simulink model "Assembly_union"  (R2020a)
settings: Solver=VariableStepAuto  StartTime=0.0  StopTime=inf  RelTol=1e-3
model workspace: external: MATLAB File A:\Usuarios\TATTO PC\Desktop\univesidad\Procesamiento video y audio\proyecto 6 intelingencia artificial\Assembly3_DataFile.m (data not in the file)
undefined symbols (not defined in the file or in its folder): smiData, X, Y, Z
libraries: neural x563, sm_lib x153, nesl_utility x4, dspstat3 x3, audiosources x1, simulink x1, dspxfrm3 x1
(part 4 of 36)

== system Assembly_union/Subsystem/Custom Neural Network6/Layer 6 ==
  "a{5} " : Inport  PortDimensions=70
      mask Display: e = 0.06;c1 = [120 230 180]/255;c2 = ([120 230 180]+0)/(256+128);c3 = ([120 230 180]+128)/(256+128);patch([0 1 1 0],[0 0 1 1],c1);patch([0 1 1 1-e 1-e 0+e],[0 0 1 1-e 0+e 0+e],c2);patch([0 0 1 1-e 0+e 0+e],[0 1 1 1-e 1-e 0+e],c3);plot([0 1 1 0 0],[0 0 1 1 0]);
  Delays 1 : Subsystem
      mask Display: e = 0.06;c1 = [120 150 230]/255;c2 = ([120 150 230]+0)/383;c3 = ([120 150 230]+128)/383;patch([0 1 1 0],[0 0 1 1],c1);patch([0 1 1 1-e 1-e 0+e],[0 0 1 1-e 0+e 0+e],c2);patch([0 0 1 1-e 0+e 0+e],[0 1 1 1-e 1-e 0+e],c3);plot([0 1 1 0 0],[0 0 1 1 0]);disp('0');
  "LW{6,5}" : Subsystem
      mask Display: e = 0.06;c1 = [120 150 230]/255;c2 = ([120 150 230]+0)/383;c3 = ([120 150 230]+128)/383;patch([0 1 1 0],[0 0 1 1],c1);patch([0 1 1 1-e 1-e 0+e],[0 0 1 1-e 0+e 0+e],c2);patch([0 0 1 1-e 0+e 0+e],[0 1 1 1-e 1-e 0+e],c3);plot([0 1 1 0 0],[0 0 1 1 0]);disp('W');
  "b{6}" : Constant  Value=[-1.485003387606178559821046292199753224849700927734375;1.4578215715256430673463228231412358582019805908203125;-1.3893651088165828166864912418532185256481170654296875;1.360850145432328961447865367517806589603424072265625;-1.3163944869522321567956169019453227519989013671875;1.2790831565414564341409686676342971622943878173828125;-1.2301069748957143001888425715151242911815643310546875;-1.2053186311808909980669568540179170668125152587890625;-1.119571343264250895543909791740588843822479248046875;-1.105184198547311869020859376178123056888580322265625;1.0496333853723898155152483013807795941829681396484375;1.0079878762454252960623080070945434272289276123046875;-0.98533438913372239920107631405699066817760467529296875;-0.94027001026555623308667009041528217494487762451171875;-0.8726319445384718154201664219726808369159698486328125;-0.85683744760427982267714241970679722726345062255859375;-0.807565898785896241207638013293035328388214111328125;0.77004429336715407572455660556443035602569580078125;0.71850134366528506379978580298484303057193756103515625;-0.647167461466730653540935236378572881221771240234375;-0.592447199662568646516547232749871909618377685546875;0.59251503759554313699453587105381302535533905029296875;-0.536368947826048714233593273092992603778839111328125;-0.5162879618890394706198776475503109395503997802734375;0.44502670176876180097025326176662929356098175048828125;-0.411594605501536758840330776365590281784534454345703125;-0.385216068976885761543371700099669396877288818359375;0.32933495686654923328973154639243148267269134521484375;0.30167834932332515673891748519963584840297698974609375;0.23611842292874019033632748687523417174816131591796875;0.1826912311398599941814069325118907727301120758056640625;-0.145968008454668396467468483024276793003082275390625;-0.10534177126921299982864610456090304069221019744873046875;0.06018886059545865141462428482554969377815723419189453125;0.007770730586208964181527125703041747328825294971466064453125;-0.003037900210818963477044096777035520062781870365142822265625;-0.050253621911659558663121316612887312658131122589111328125;0.09786422466005463560723143245922983624041080474853515625;0.1510481711326792375604810558797908015549182891845703125;-0.1959526938701692533317810784865287132561206817626953125;-0.2351624924981109698851611256031901575624942779541015625;-0.277950698490396330697649318608455359935760498046875;-0.336603419162789518903622365542105399072170257568359375;-0.35305899148826125344413640050333924591541290283203125;-0.413619138650432704995552057880559004843235015869140625;-0.444163369013349740299645418417640030384063720703125;0.484800773696828446457374184319633059203624725341796875;0.55997085323872630713282205761061049997806549072265625;0.5889112097013391444733088064822368323802947998046875;0.6266854932690610890944071798003278672695159912109375;0.66414649891511590151793598124640993773937225341796875;0.70284249294120770823468546950607560575008392333984375;0.748702178371122517575031451997347176074981689453125;0.80946782172921671882903638106654398143291473388671875;-0.84566429400031228880152411875315010547637939453125;-0.88906859934408632994973231689073145389556884765625;-0.90484521568163334137580022797919809818267822265625;-0.97417279264519651693632340538897551596164703369140625;-1.023583515821328671080436834017746150493621826171875;1.0530542658285824142438968920032493770122528076171875;-1.091398208237234879192101288936100900173187255859375;1.141249173995749988108627803740091621875762939453125;-1.1619243888892019089809082288411445915699005126953125;-1.2241454031893457266022551266360096633434295654296875;1.2750005254271881138805611044517718255519866943359375;1.32597692828655322472286570700816810131072998046875;1.3199231160172217869330779649317264556884765625;1.404688225611195218078819380025379359722137451171875;1.44054888145474624394637430668808519840240478515625;-1.483986405440906874986239927238784730434417724609375]
      mask Display: e = 0.06;c1 = [120 150 230]/255;c2 = ([120 150 230]+0)/383;c3 = ([120 150 230]+128)/383;patch([0 1 1 0],[0 0 1 1],c1);patch([0 1 1 1-e 1-e 0+e],[0 0 1 1-e 0+e 0+e],c2);patch([0 0 1 1-e 0+e 0+e],[0 1 1 1-e 1-e 0+e],c3);plot([0 1 1 0 0],[0 0 1 1 0]);disp('b');
  netsum : Sum  Inputs=2  InputSameDT=on  SaturateOnIntegerOverflow=on  OutDataTypeStr=Inherit: Same as first input
      mask Display: e = 0.06;c1 = [120 150 230]/255;c2 = ([120 150 230]+0)/383;c3 = ([120 150 230]+128)/383;patch([0 1 1 0],[0 0 1 1],c1);patch([0 1 1 1-e 1-e 0+e],[0 0 1 1-e 0+e 0+e],c2);patch([0 0 1 1-e 0+e 0+e],[0 1 1 1-e 1-e 0+e],c3);plot([0 1 1 0 0],[0 0 1 1 0]);disp('+');
  tansig : neural/Transfer Functions/tansig
  "a{6}" : Outport  InitialOutput=[0;0;0;0;0;0;0;0;0;0;0;0;0;0;0;0;0;0;0;0;0;0;0;0;0;0;0;0;0;0;0;0;0;0;0;0;0;0;0;0;0;0;0;0;0;0;0;0;0;0;0;0;0;0;0;0;0;0;0;0;0;0;0;0;0;0;0;0;0;0]
      mask Display: e = 0.06;c1 = [120 230 180]/255;c2 = ([120 230 180]+0)/(256+128);c3 = ([120 230 180]+128)/(256+128);patch([0 1 1 0],[0 0 1 1],c1);patch([0 1 1 1-e 1-e 0+e],[0 0 1 1-e 0+e 0+e],c2);patch([0 0 1 1-e 0+e 0+e],[0 1 1 1-e 1-e 0+e],c3);plot([0 1 1 0 0],[0 0 1 1 0]);
  wires:
  "a{5} "/1 -> Delays 1/1("p{6}")
  Delays 1/1("pd{6,5}") -> "LW{6,5}"/1("ad{6,5}")
  "LW{6,5}"/1("lz{6,5}") -> netsum/1
  "b{6}"/1 -> netsum/2
  netsum/1 -> tansig/1
  tansig/1 -> "a{6}"/1

== system Assembly_union/Subsystem/Custom Neural Network6/Layer 7 ==
  "a{6} " : Inport  PortDimensions=70
      mask Display: e = 0.06;c1 = [120 230 180]/255;c2 = ([120 230 180]+0)/(256+128);c3 = ([120 230 180]+128)/(256+128);patch([0 1 1 0],[0 0 1 1],c1);patch([0 1 1 1-e 1-e 0+e],[0 0 1 1-e 0+e 0+e],c2);patch([0 0 1 1-e 0+e 0+e],[0 1 1 1-e 1-e 0+e],c3);plot([0 1 1 0 0],[0 0 1 1 0]);
  Delays 1 : Subsystem
      mask Display: e = 0.06;c1 = [120 150 230]/255;c2 = ([120 150 230]+0)/383;c3 = ([120 150 230]+128)/383;patch([0 1 1 0],[0 0 1 1],c1);patch([0 1 1 1-e 1-e 0+e],[0 0 1 1-e 0+e 0+e],c2);patch([0 0 1 1-e 0+e 0+e],[0 1 1 1-e 1-e 0+e],c3);plot([0 1 1 0 0],[0 0 1 1 0]);disp('0');
  "LW{7,6}" : Subsystem
      mask Display: e = 0.06;c1 = [120 150 230]/255;c2 = ([120 150 230]+0)/383;c3 = ([120 150 230]+128)/383;patch([0 1 1 0],[0 0 1 1],c1);patch([0 1 1 1-e 1-e 0+e],[0 0 1 1-e 0+e 0+e],c2);patch([0 0 1 1-e 0+e 0+e],[0 1 1 1-e 1-e 0+e],c3);plot([0 1 1 0 0],[0 0 1 1 0]);disp('W');
  "b{7}" : Constant  Value=[-1.4767621523240166414581153730978257954120635986328125;1.444049296004457527686781759257428348064422607421875;-1.4013145988464714708499059270252473652362823486328125;1.3335134565628778968715550945489667356014251708984375;1.3236197336460235884914027337799780070781707763671875;1.27579077866800094653854102944023907184600830078125;-1.21593386784343948647801880724728107452392578125;1.178120321207556830955809346050955355167388916015625;-1.12775361173192489872008081874810159206390380859375;1.078399371995239608423844401841051876544952392578125;-1.0560677697311307010608061318635009229183197021484375;1.0272419780436761183040061951032839715480804443359375;0.99828915385229344270356932611321099102497100830078125;-0.8858404721323822617051746419747360050678253173828125;-0.8576324002365949272785883295000530779361724853515625;0.8292697266285691259923851248458959162235260009765625;-0.8083178375879727095565385752706788480281829833984375;0.7069678528848524212691017964971251785755157470703125;-0.691934107202713644113600821583531796932220458984375;-0.62273911879922361212180703660123981535434722900390625;-0.61509936217620875265055246927659027278423309326171875;0.57882003721991981404215721340733580291271209716796875;0.539682981503778247400759937590919435024261474609375;-0.4993444993130979892015375298797152936458587646484375;0.469344644639037744671128393747494556009769439697265625;0.4214914724469507323334482862264849245548248291015625;-0.37938438865782397879655718497815541923046112060546875;-0.304543847702456293990991298414883203804492950439453125;0.284100250478663551856328695066622458398342132568359375;0.2391032035570020142234426430150051601231098175048828125;-0.1971118230385970060414280169425182975828647613525390625;-0.1768708078998612320820171817103982903063297271728515625;0.11242682486000869779285693539350177161395549774169921875;-0.06773328044365271860538513237770530395209789276123046875;0.01283256275473169949474794293564627878367900848388671875;0.052509615656154202956162890814084676094353199005126953125;0.056595446575947082334945292814154527150094509124755859375;0.0957661037569482453957192547022714279592037200927734375;0.1710599168838210226706308958455338142812252044677734375;-0.2004174313203110902037451523938216269016265869140625;0.2335509297283305529813191014909534715116024017333984375;0.310312095338587445869649172891513444483280181884765625;0.305696289894037409595739518408663570880889892578125;-0.36359794360045449845841858405037783086299896240234375;0.40952848771876404487812806110014207661151885986328125;0.438142211964403560653380509393173269927501678466796875;-0.53602802650183123400751128428964875638484954833984375;-0.5537352484590680745668578310869634151458740234375;0.5633847814036225809530833430471830070018768310546875;-0.60758518515698900497312706647790037095546722412109375;0.67224387508036897997953929007053375244140625;0.7521169924806463402688905262039043009281158447265625;-0.75404805176073186334662068475154228508472442626953125;0.78505703476111332594911118576419539749622344970703125;0.84022623832228882090333854648633860051631927490234375;0.89421096481471218364589503835304640233516693115234375;0.92810077829095971591044644810608588159084320068359375;-0.9541226123161259398131051057134754955768585205078125;1.008752849302839482703575413324870169162750244140625;-1.0517509919543404084407711707171984016895294189453125;1.0948916566899244973143368042656220495700836181640625;-1.122592887192439103927199539612047374248504638671875;-1.173968638316350787675901301554404199123382568359375;-1.213892733483060926147345526260323822498321533203125;1.2715677661036901557878309176885522902011871337890625;1.3291196102867590678187070807325653731822967529296875;-1.3539816759775289423117783371708355844020843505859375;-1.4025819142239408510164366816752590239048004150390625;1.4116364927836217990630984786548651754856109619140625;1.501802361522918349834299078793264925479888916015625]
      mask Display: e = 0.06;c1 = [120 150 230]/255;c2 = ([120 150 230]+0)/383;c3 = ([120 150 230]+128)/383;patch([0 1 1 0],[0 0 1 1],c1);patch([0 1 1 1-e 1-e 0+e],[0 0 1 1-e 0+e 0+e],c2);patch([0 0 1 1-e 0+e 0+e],[0 1 1 1-e 1-e 0+e],c3);plot([0 1 1 0 0],[0 0 1 1 0]);disp('b');
  netsum : Sum  Inputs=2  InputSameDT=on  SaturateOnIntegerOverflow=on  OutDataTypeStr=Inherit: Same as first input
      mask Display: e = 0.06;c1 = [120 150 230]/255;c2 = ([120 150 230]+0)/383;c3 = ([120 150 230]+128)/383;patch([0 1 1 0],[0 0 1 1],c1);patch([0 1 1 1-e 1-e 0+e],[0 0 1 1-e 0+e 0+e],c2);patch([0 0 1 1-e 0+e 0+e],[0 1 1 1-e 1-e 0+e],c3);plot([0 1 1 0 0],[0 0 1 1 0]);disp('+');
  tansig : neural/Transfer Functions/tansig
  "a{7}" : Outport  InitialOutput=[0;0;0;0;0;0;0;0;0;0;0;0;0;0;0;0;0;0;0;0;0;0;0;0;0;0;0;0;0;0;0;0;0;0;0;0;0;0;0;0;0;0;0;0;0;0;0;0;0;0;0;0;0;0;0;0;0;0;0;0;0;0;0;0;0;0;0;0;0;0]
      mask Display: e = 0.06;c1 = [120 230 180]/255;c2 = ([120 230 180]+0)/(256+128);c3 = ([120 230 180]+128)/(256+128);patch([0 1 1 0],[0 0 1 1],c1);patch([0 1 1 1-e 1-e 0+e],[0 0 1 1-e 0+e 0+e],c2);patch([0 0 1 1-e 0+e 0+e],[0 1 1 1-e 1-e 0+e],c3);plot([0 1 1 0 0],[0 0 1 1 0]);
  wires:
  "a{6} "/1 -> Delays 1/1("p{7}")
  Delays 1/1("pd{7,6}") -> "LW{7,6}"/1("ad{7,6}")
  "LW{7,6}"/1("lz{7,6}") -> netsum/1
  "b{7}"/1 -> netsum/2
  netsum/1 -> tansig/1
  tansig/1 -> "a{7}"/1

== system Assembly_union/Subsystem/Custom Neural Network6/Layer 8 ==
  "a{7} " : Inport  PortDimensions=70
      mask Display: e = 0.06;c1 = [120 230 180]/255;c2 = ([120 230 180]+0)/(256+128);c3 = ([120 230 180]+128)/(256+128);patch([0 1 1 0],[0 0 1 1],c1);patch([0 1 1 1-e 1-e 0+e],[0 0 1 1-e 0+e 0+e],c2);patch([0 0 1 1-e 0+e 0+e],[0 1 1 1-e 1-e 0+e],c3);plot([0 1 1 0 0],[0 0 1 1 0]);
  Delays 1 : Subsystem
      mask Display: e = 0.06;c1 = [120 150 230]/255;c2 = ([120 150 230]+0)/383;c3 = ([120 150 230]+128)/383;patch([0 1 1 0],[0 0 1 1],c1);patch([0 1 1 1-e 1-e 0+e],[0 0 1 1-e 0+e 0+e],c2);patch([0 0 1 1-e 0+e 0+e],[0 1 1 1-e 1-e 0+e],c3);plot([0 1 1 0 0],[0 0 1 1 0]);disp('0');
  "LW{8,7}" : Subsystem
      mask Display: e = 0.06;c1 = [120 150 230]/255;c2 = ([120 150 230]+0)/383;c3 = ([120 150 230]+128)/383;patch([0 1 1 0],[0 0 1 1],c1);patch([0 1 1 1-e 1-e 0+e],[0 0 1 1-e 0+e 0+e],c2);patch([0 0 1 1-e 0+e 0+e],[0 1 1 1-e 1-e 0+e],c3);plot([0 1 1 0 0],[0 0 1 1 0]);disp('W');
  "b{8}" : Constant  Value=[1.4870503804997989849567829878651537001132965087890625;-1.3951167688820780288239120636717416346073150634765625;-1.327618360170772948691819692612625658512115478515625;1.306601799763808191556790916365571320056915283203125;1.2663434339955046414871731030871160328388214111328125;1.190710745246216450965448530041612684726715087890625;-1.146077751003579781041707974509336054325103759765625;1.1207008038467944910365758914849720895290374755859375;-1.076304867027505718368729503708891570568084716796875;-1.0124811514544884705202321129036135971546173095703125;0.99231961835159199214473346728482283651828765869140625;-0.94089816984124585719229116875794716179370880126953125;-0.87244570582967828631382189996656961739063262939453125;0.8277766961789716493314017498050816357135772705078125;0.780486675323220691069536769646219909191131591796875;-0.7615131860318140599730440953862853348255157470703125;-0.68486451279397864144726781887584365904331207275390625;0.62709947678303412654798876246786676347255706787109375;-0.64579718495621174501053474159562028944492340087890625;0.55706567783365013024621248405310325324535369873046875;-0.5049344991792865666724310358404181897640228271484375;0.472820940457257699041093701453064568340778350830078125;0.429017711810034507724509467152529396116733551025390625;0.3446190033229241667100950508029200136661529541015625;-0.364759573889755939202217405181727372109889984130859375;-0.27309037684208214979975082314922474324703216552734375;-0.225284470232680777979084041362511925399303436279296875;-0.1621828502858713993983741374904639087617397308349609375;-0.10689277157941645679528619439224712550640106201171875;-0.103259609314033273808064450349775142967700958251953125;0.03884901518316140334174946247003390453755855560302734375;0.0005746932371042067465294334027703371248207986354827880859375;0.075747738710083278856899369202437810599803924560546875;0.133160366097609561553127832667087204754352569580078125;-0.1282758525387227288572233874219818972051143646240234375;0.228615838596995579745652094061370007693767547607421875;0.262002979551309633787781194769195280969142913818359375;0.29756545401996914446129949283204041421413421630859375;0.331290148292351760428431362015544436872005462646484375;-0.36134855665765364118868774312431924045085906982421875;-0.431312721022454492736386555407079868018627166748046875;-0.507788270686636789008616688079200685024261474609375;-0.489747930073772985704039228949113748967647552490234375;-0.542204463994927277070701165939681231975555419921875;0.62752050227328159959228059960878454148769378662109375;-0.6472957097511076174356503543094731867313385009765625;-0.70956954367255853366458495656843297183513641357421875;-0.77245364970295238293829243048094213008880615234375;-0.7991690658306220829132371363812126219272613525390625;-0.819577914249400851787186184083111584186553955078125;-0.85887340289468838694375563136418350040912628173828125;0.93052457276767863714184159107389859855175018310546875;1.008288804793448623087215310079045593738555908203125;1.02744932602150829126230746624059975147247314453125;1.0679041121665824309872050434933044016361236572265625;-1.1188048689090825948966312353149987757205963134765625;-1.1842143338128472418446790470625273883342742919921875;1.227123639146034062008538967347703874111175537109375;1.273134746498172820139416216989047825336456298828125;-1.3148719450415471410309464772581122815608978271484375;1.3679120366305383971194942205329425632953643798828125;1.3820408132081738461494069269974716007709503173828125;-1.4138192314707989094557660791906528174877166748046875]
      mask Display: e = 0.06;c1 = [120 150 230]/255;c2 = ([120 150 230]+0)/383;c3 = ([120 150 230]+128)/383;patch([0 1 1 0],[0 0 1 1],c1);patch([0 1 1 1-e 1-e 0+e],[0 0 1 1-e 0+e 0+e],c2);patch([0 0 1 1-e 0+e 0+e],[0 1 1 1-e 1-e 0+e],c3);plot([0 1 1 0 0],[0 0 1 1 0]);disp('b');
  netsum : Sum  Inputs=2  InputSameDT=on  SaturateOnIntegerOverflow=on  OutDataTypeStr=Inherit: Same as first input
      mask Display: e = 0.06;c1 = [120 150 230]/255;c2 = ([120 150 230]+0)/383;c3 = ([120 150 230]+128)/383;patch([0 1 1 0],[0 0 1 1],c1);patch([0 1 1 1-e 1-e 0+e],[0 0 1 1-e 0+e 0+e],c2);patch([0 0 1 1-e 0+e 0+e],[0 1 1 1-e 1-e 0+e],c3);plot([0 1 1 0 0],[0 0 1 1 0]);disp('+');
  tansig : neural/Transfer Functions/tansig
  "a{8}" : Outport  InitialOutput=[0;0;0;0;0;0;0;0;0;0;0;0;0;0;0;0;0;0;0;0;0;0;0;0;0;0;0;0;0;0;0;0;0;0;0;0;0;0;0;0;0;0;0;0;0;0;0;0;0;0;0;0;0;0;0;0;0;0;0;0;0;0;0]
      mask Display: e = 0.06;c1 = [120 230 180]/255;c2 = ([120 230 180]+0)/(256+128);c3 = ([120 230 180]+128)/(256+128);patch([0 1 1 0],[0 0 1 1],c1);patch([0 1 1 1-e 1-e 0+e],[0 0 1 1-e 0+e 0+e],c2);patch([0 0 1 1-e 0+e 0+e],[0 1 1 1-e 1-e 0+e],c3);plot([0 1 1 0 0],[0 0 1 1 0]);
  wires:
  "a{7} "/1 -> Delays 1/1("p{8}")
  Delays 1/1("pd{8,7}") -> "LW{8,7}"/1("ad{8,7}")
  "LW{8,7}"/1("lz{8,7}") -> netsum/1
  "b{8}"/1 -> netsum/2
  netsum/1 -> tansig/1
  tansig/1 -> "a{8}"/1

== system Assembly_union/Subsystem/Custom Neural Network6/Process Input 1 ==
  x : Inport  PortDimensions=63
      mask Display: e = 0.06;c1 = [120 230 180]/255;c2 = ([120 230 180]+0)/(256+128);c3 = ([120 230 180]+128)/(256+128);patch([0 1 1 0],[0 0 1 1],c1);patch([0 1 1 1-e 1-e 0+e],[0 0 1 1-e 0+e 0+e],c2);patch([0 0 1 1-e 0+e 0+e],[0 1 1 1-e 1-e 0+e],c3);plot([0 1 1 0 0],[0 0 1 1 0]);
  mapminmax : neural/Processing Functions/mapminmax  xmin=[8.1803971064829148112301305043e-07;1.09299653407800229163848032554e-06;1.5927335694390287421670724527e-06;1.67220969003334483195377505906e-07;1.59359277813771457052113324215e-06;8.13845157553307709175820575109e-07;9.69952896519324843461269843037e-07;1.20431645734910159755174860474e-06;8.52603689316611955066442258416e-07;6.40588731482611470838945105094e-07;3.00998118272467163659842021364e-07;5.35031323872808453076890550931e-07;3.47608539059446699199889228848e-07;8.22257677446769589023952296697e-07;5.82173566500407632774781018642e-08;1.25416314625186030249910477952e-06;4.32102595749552161881701329779e-07;3.5522490804120083726622722313e-07;2.26336830983664327188051518594e-07;9.5542644693102875605829685246e-07;4.50121359260190538159303666466e-07;6.95553929115588461581237700315e-07;8.62880737022771244770509135175e-07;5.65407781661879991484166447374e-07;8.34371642623087653566223663437e-07;3.61109309634215936156463946927e-07;2.13087430503505320907842147081e-07;4.1623754623760123074537411493e-07;5.84691285052120298880407815029e-07;9.18221769995487102182925255242e-08;4.37679765709770867931319333899e-07;3.19719425702207398420299361286e-07;1.02291856756473327088902570275e-06;1.10371016863100540161390233918e-06;8.06674870577285928609050091875e-07;9.3129097249289943253778515514e-07;8.90531037018537233893803860968e-07;2.96843013098934481307249926355e-07;4.55314794206472742894875084529e-07;1.34920881415412646758117658913e-06;7.26556782948189951859552238034e-07;4.29168750842285899479267670051e-07;7.38537900894562454111953644226e-07;7.80541969953873840776757946774e-07;1.16734113261423605269260887762e-06;4.23195008766250489867506538733e-07;5.81844754352267676090842106473e-07;2.76515490764371361414377401347e-07;6.60468671121587166424190748493e-07;7.27937702988538397966538241041e-07;5.46961091767035564959538625207e-07;7.7190380483956900376109723852e-07;4.48245500773484959207274870574e-07;4.30959829018163090417917280434e-07;7.36732139598862547792798745327e-07;2.94957337179709438628263679788e-07;2.74783783678781645588189760238e-07;2.42297545439280319989032311603e-07;3.63591352149734483665540841005e-07;6.36721919052513792308559213012e-07;9.67374979918825999083975553106e-07;4.62822630279331582971240029514e-07;2.7066816670529611054546448301e-07]  xmax=[0.0102756076840403200167717301383;0.013023392523126703368419043727;0.0146158383882840654105494948567;0.0210163578378903259658017077527;0.03488982277329762821116432292;0.207238735537912693862594437633;0.0464074339773329416769520605612;0.0363412271337583137054139115207;0.0888454585993229684071081919683;0.112098958074779667115628001284;0.0586766281671914011197621618976;0.275714654059784625150797410242;0.122224659796826062851948790922;0.0462519395167219626863186476839;0.0302811796813280340034957305306;0.0635254794406884398805246405573;0.426615569075903255935600100202;0.0865855147919272621903630238194;0.03913849772467659776653547965;0.0171971109372166600093301269681;0.0163267591030779486704904712724;0.0139947771098405185363766634055;0.00911046623738340048681561000876;0.0162495637059484436537371010445;0.0496528828419279325001589597832;0.00976999060409301962881745140521;0.00678022972009770501927716779278;0.00762090784752180155220413482198;0.006933111036987914081730632887;0.0140379040348495125190009247262;0.0212938364023411777492533758505;0.00607395615112893243192626613336;0.00550955974730480985829261797448;0.00715673637984898074193562678147;0.00704443581180925516849189449431;0.00538966574981211612310749714538;0.00584260678705436197616363003249;0.00769139756809718994068347797111;0.0108124275361523025651422358351;0.0276429089812400656522850539432;0.0161504471763809012707646672879;0.00555745780595186950057140506942;0.011244510411302944055678132429;0.00341307658293585770153955039063;0.00673972668674419246592766086223;0.0032949861814823831231147099885;0.00344534876455327744582124438466;0.0156322857596569303462175071218;0.028690404653391246569960060242;0.019132155760524040960524061461;0.00300509310001731812581060587775;0.00452842256731891563276137802063;0.00426991088912471832006456651243;0.0115193530202442329102296980636;0.0189678851722498015286433314941;0.0799426759657599766972779775642;0.0222892606548130145505126620264;0.0161594698456761394489422656306;0.0110505555775375057664389188972;0.00641505193152908190917793618269;0.00601988898151582969842099402058;0.00582167039613013317933543078198;0.0259507732823324871462844498637]  ymin=-1  ymax=1
  p : Outport  PortDimensions=63
      mask Display: e = 0.06;c1 = [120 230 180]/255;c2 = ([120 230 180]+0)/(256+128);c3 = ([120 230 180]+128)/(256+128);patch([0 1 1 0],[0 0 1 1],c1);patch([0 1 1 1-e 1-e 0+e],[0 0 1 1-e 0+e 0+e],c2);patch([0 0 1 1-e 0+e 0+e],[0 1 1 1-e 1-e 0+e],c3);plot([0 1 1 0 0],[0 0 1 1 0]);
  wires:
  x/1 -> mapminmax/1
  mapminmax/1 -> p/1

== system Assembly_union/Subsystem/Custom Neural Network6/Process Output 1 ==
  a : Inport  PortDimensions=63
      mask Display: e = 0.06;c1 = [120 230 180]/255;c2 = ([120 230 180]+0)/(256+128);c3 = ([120 230 180]+128)/(256+128);patch([0 1 1 0],[0 0 1 1],c1);patch([0 1 1 1-e 1-e 0+e],[0 0 1 1-e 0+e 0+e],c2);patch([0 0 1 1-e 0+e 0+e],[0 1 1 1-e 1-e 0+e],c3);plot([0 1 1 0 0],[0 0 1 1 0]);
  mapminmax_reverse : neural/Processing Functions/mapminmax_reverse  xmin=[0;0;0;0;0;0;0;0;0;0;0;0;0;0;0;0;0;0;0;0;0;0;0;0;0;0;0;0;0;0;0;0;0;0;0;0;0;0;0;0;0;0;0;0;0;0;0;0;0;0;0;0;0;0;0;0;0;0;0;0;0;0;0]  xmax=[8;8;8;8;8;8;8;8;8;8;8;8;8;8;8;8;8;8;8;8;8;8;8;8;8;8;8;8;8;8;8;8;8;8;8;8;8;8;8;8;8;8;8;8;8;8;8;8;8;8;8;8;8;8;8;8;8;8;8;8;8;8;8]  ymin=-1  ymax=1
  y : Outport  PortDimensions=63
      mask Display: e = 0.06;c1 = [120 230 180]/255;c2 = ([120 230 180]+0)/(256+128);c3 = ([120 230 180]+128)/(256+128);patch([0 1 1 0],[0 0 1 1],c1);patch([0 1 1 1-e 1-e 0+e],[0 0 1 1-e 0+e 0+e],c2);patch([0 0 1 1-e 0+e 0+e],[0 1 1 1-e 1-e 0+e],c3);plot([0 1 1 0 0],[0 0 1 1 0]);
  wires:
  a/1 -> mapminmax_reverse/1
  mapminmax_reverse/1 -> y/1

== system Assembly_union/Subsystem/Custom Neural Network6/Layer 1/Delays 1 ==
  "p{1}" : Inport  PortDimensions=63
      mask Display: e = 0.06;c1 = [120 230 180]/255;c2 = ([120 230 180]+0)/(256+128);c3 = ([120 230 180]+128)/(256+128);patch([0 1 1 0],[0 0 1 1],c1);patch([0 1 1 1-e 1-e 0+e],[0 0 1 1-e 0+e 0+e],c2);patch([0 0 1 1-e 0+e 0+e],[0 1 1 1-e 1-e 0+e],c3);plot([0 1 1 0 0],[0 0 1 1 0]);
  mux : Mux  Inputs=1
      mask Display: e = 0.06;c1 = [120 150 230]/255;c2 = ([120 150 230]+0)/383;c3 = ([120 150 230]+128)/383;patch([0 1 1 0],[0 0 1 1],c1);patch([0 1 1 1-e 1-e 0+e],[0 0 1 1-e 0+e 0+e],c2);patch([0 0 1 1-e 0+e 0+e],[0 1 1 1-e 1-e 0+e],c3);plot([0 1 1 0 0],[0 0 1 1 0]);disp('Mux')
  "pd{1,1}" : Outport
      mask Display: e = 0.06;c1 = [120 230 180]/255;c2 = ([120 230 180]+0)/(256+128);c3 = ([120 230 180]+128)/(256+128);patch([0 1 1 0],[0 0 1 1],c1);patch([0 1 1 1-e 1-e 0+e],[0 0 1 1-e 0+e 0+e],c2);patch([0 0 1 1-e 0+e 0+e],[0 1 1 1-e 1-e 0+e],c3);plot([0 1 1 0 0],[0 0 1 1 0]);
  wires:
  "p{1}"/1 -> mux/1
  mux/1 -> "pd{1,1}"/1
